simulink model "model0"  (R2020a)
settings: Solver=FixedStepDiscrete  StartTime=0.0  StopTime=10.0  FixedStep=0.1  RelTol=1e-3
settings Model: Creator=gmcvi  LastModifiedBy=gmcvi
settings SolverCC: AutoInsertRateTranBlk=on
settings OptimizationCC: DefaultParameterBehavior=Inlined  EnhancedBackFolding=on  PassReuseOutputArgsAs=Individual arguments  ZeroExternalMemoryAtStartup=off  ZeroInternalMemoryAtStartup=off  OptimizeBlockOrder=speed  DifferentSizesBufferReuse=on  OptimizationCustomize=off  EfficientTunableParamExpr=on
settings DebuggingCC: ParameterTunabilityLossMsg=error
settings SFSimCC: MATLABDynamicMemAlloc=off
settings RTWCC: SystemTargetFile=ert.tlc  GenCodeOnly=on  TemplateMakefile=ert_default_tmf  Toolchain=MinGW64 | gmake (64-bit Windows)  TargetLang=C++
settings CodeAppCC: ForceParamTrailComments=on  IgnoreCustomStorageClasses=off  OperatorAnnotations=on  SimulinkDataObjDesc=on  SFDataObjDesc=on  InsertBlockDesc=on
settings ERTTargetCC: TargetLangStandard=C++03 (ISO)  GenerateSampleERTMain=on  InlinedParameterPlacement=NonHierarchical  RootIOFormat=Structure reference  ERTCustomFileTemplate=example_file_process.tlc

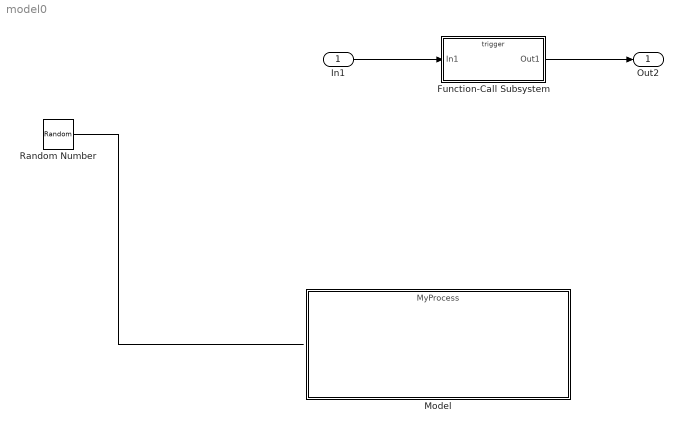
== system model0 ==
  In1 : Inport
  Function-Call Subsystem : Subsystem  TreatAsAtomicUnit=on
  Model : ModelReference  ModelNameDialog=MyProcess.slx  SimulationMode=Normal  ModelReferenceVersion=1.7
  Random Number : RandomNumber  SampleTime=1.3
  Out2 : Outport
  wires:
  Random Number/1 -> ?
  Function-Call Subsystem/1(Out1) -> Out2/1
  In1/1 -> Function-Call Subsystem/1(In1)

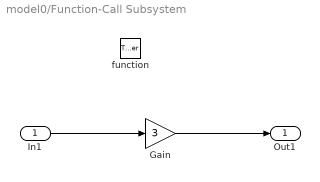
== system model0/Function-Call Subsystem ==
  In1 : Inport
  function : TriggerPort  TriggerType=function-call  IsSimulinkFunction=on  FunctionName=fun  FunctionVisibility=scoped  VariantControl=Variant
  Gain : Gain  Gain=3
  Out1 : Outport
  wires:
  In1/1 -> Gain/1
  Gain/1 -> Out1/1
